simulink model "First_and_Second_SystemOrder"  (R2021a)
settings: Solver=VariableStepAuto  StartTime=0.0  StopTime=10.0  RelTol=1e-3
settings Model: Creator=lenovo  LastModifiedBy=lenovo

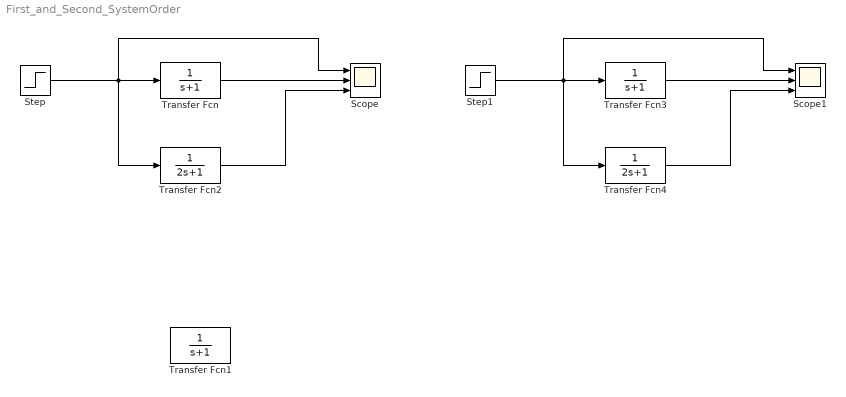
== system First_and_Second_SystemOrder ==
  Scope : Scope  NumInputPorts=3
  Scope1 : Scope  NumInputPorts=3
  Step : Step  SampleTime=0
  Step1 : Step  SampleTime=0
  Transfer Fcn : TransferFcn  Denominator=[1 1]
  Transfer Fcn1 : TransferFcn  Denominator=[1 1]
  Transfer Fcn2 : TransferFcn  Denominator=[2 1]
  Transfer Fcn3 : TransferFcn  Denominator=[1 1]
  Transfer Fcn4 : TransferFcn  Denominator=[2 1]
  wires:
  Step/1 -> Transfer Fcn2/1, Scope/1, Transfer Fcn/1
  Transfer Fcn/1 -> Scope/2
  Transfer Fcn2/1 -> Scope/3
  Transfer Fcn4/1 -> Scope1/3
  Transfer Fcn3/1 -> Scope1/2
  Step1/1 -> Transfer Fcn3/1, Scope1/1, Transfer Fcn4/1
